simulink model "bu_abslut125_romvect_float"  (R2021b)
(part 3 of 8)

  AddSub121/1 -> Mux119/3
  Delay489/1 -> Relational184/1, Delay492/1
  AddSub163/1 -> Mux170/3
  Mux144/1 -> AddSub148/1, Delay376/1
  Delay586/1 -> Mux114/2
  Delay397/1 -> Mux160/1
  Delay542/1 -> Mux124/2
  Mux126/1 -> AddSub183/1, Delay245/1
  Delay529/1 -> Mux181/2
  Delay525/1 -> Mux169/2
  Delay550/1 -> Mux127/2
  Delay354/1 -> Mux152/2
  Delay248/1 -> Mux141/2
  Relational154/1 -> Delay350/1
  Relational199/1 -> Delay442/1
  AddSub181/1 -> Mux178/3
  Delay458/1 -> Mux102/1
  Mux95/1 -> AddSub99/1, Delay209/1
  Delay377/1 -> Delay378/1, Relational148/1
  Delay388/1 -> Relational160/1, Delay344/1
  AddSub124/1 -> Mux122/3
  Relational189/1 -> Delay504/1
  logi_b69/1 -> Relational145/2, Relational151/2
  Delay362/1 -> Mux154/2
  Delay378/1 -> Delay381/1, Relational149/1
  Delay473/1 -> Mux183/1
  AddSub188/1 -> Mux187/3
  Delay423/1 -> Mux163/2
  AddSub98/1 -> Mux95/3
  Mux162/1 -> AddSub165/1, Delay491/1
  Mux173/1 -> AddSub176/1, Delay469/1
  logi_b75/1 -> Relational153/2, Relational159/2
  Delay428/1 -> Relational101/1, Delay432/1
  Relational150/1 -> Delay386/1
  Delay480/1 -> Mux177/2
  Delay585/1 -> Mux114/1
  logi_b78/1 -> Relational177/2, Relational192/2
  Delay570/1 -> Delay573/1, Relational136/1
  Mux182/1 -> AddSub192/1, Delay411/1
  AddSub195/1 -> Mux163/3
  Relational115/1 -> Delay590/1
  Relational137/1 -> Delay578/1
  Relational185/1 -> Delay446/1
  Delay517/1 -> Mux120/2
  logi_b71/1 -> Relational147/2, Relational155/2
  Delay590/1 -> Mux115/1
  Delay210/1 -> Mux130/1
  Mux153/1 -> AddSub156/1, Delay362/1
  Delay415/1 -> Delay436/1, Relational197/1
  Delay511/1 -> Relational167/1, Delay514/1
  Delay484/1 -> Mux183/2
  Delay492/1 -> Relational186/1, Delay496/1
  Relational171/1 -> Delay527/1
  Delay557/1 -> Mux95/1
  AddSub106/1 -> Mux102/3
  Delay358/1 -> Mux153/2
  Delay589/1 -> Delay592/1, Relational116/1
  Relational174/1 -> Delay429/1
  Delay350/1 -> Mux151/1
  AddSub200/1 -> Mux197/3
  Delay420/1 -> Delay424/1, Relational200/1
  logi_b76/1 -> Relational160/2, Relational161/2
  Relational151/1 -> Delay340/1
  logi_b70/1 -> Relational146/2, Relational154/2
  AddSub107/1 -> Mux103/3
  logi_b67/1 -> Relational140/2, Relational142/2
  Delay367/1 -> Mux156/1
  Mux168/1 -> AddSub171/1, Delay525/1
  AddSub154/1 -> Mux149/3
  Relational146/1 -> Delay372/1
  Delay442/1 -> Mux197/1
  Mux133/1 -> AddSub135/1, Delay572/1
  Delay414/1 -> Mux193/2
  Mux170/1 -> AddSub173/1, Delay419/1
  Relational147/1 -> Delay375/1
  Mux104/1 -> AddSub101/1, Delay558/1
  AddSub180/1 -> Mux190/3
  Mux192/1 -> Delay418/1, AddSub104/1
  Mux113/1 -> AddSub117/1, Delay586/1
  AddSub134/1 -> Mux133/3
  Delay583/1 -> Mux113/2
  Delay569/1 -> Mux133/2
  AddSub118/1 -> Mux115/3
  Relational176/1 -> Delay487/1
  Delay559/1 -> Relational132/1, Delay562/1
  Mux131/1 -> AddSub132/1, Delay564/1
  Delay457/1 -> Relational175/1, Delay460/1
  Relational112/1 -> Delay224/1
  Delay436/1 -> Relational198/1, Delay441/1
  Delay394/1 -> Mux164/2
  Relational133/1 -> Delay563/1
  Delay591/1 -> Mux115/2
  Delay500/1 -> Delay503/1, Relational189/1
  Delay496/1 -> Delay497/1, Relational187/1
  Delay587/1 -> Delay589/1, Relational115/1
  AddSub136/1 -> Mux135/3
  logi_b92/1 -> Relational173/2, Relational190/2
  Delay515/1 -> Mux167/1
  Delay459/1 -> Mux102/2
  Relational162/1 -> Delay402/1
  Relational144/1 -> Delay332/1
  Mux187/1 -> AddSub189/1, Delay505/1
  Delay488/1 -> Mux162/2
  Delay223/1 -> Delay581/1, Relational112/1
  Relational113/1 -> Delay582/1
  AddSub123/1 -> Mux121/3
  Delay467/1 -> Relational178/1, Delay470/1
  Mux156/1 -> AddSub160/1, Delay343/1
  Delay222/1 -> Delay547/1, Relational37/1
  Delay553/1 -> Mux119/1
  Delay594/1 -> Mux116/2
  Delay439/1 -> Relational196/1, Delay462/1
  Relational193/1 -> Delay406/1
  AddSub116/1 -> Mux113/3
  Delay592/1 -> Delay595/1, Relational117/1
  Relational121/1 -> Delay553/1
  Relational130/1 -> Delay588/1
  Relational136/1 -> Delay574/1
  Delay462/1 -> Relational122/1, Delay495/1
  Mux197/1 -> AddSub138/1, Delay234/1
  Mux184/1 -> AddSub185/1, Delay494/1
  Mux130/1 -> AddSub141/1, Delay253/1
  Mux146/1 -> AddSub151/1, Delay384/1
  Mux191/1 -> Delay414/1, AddSub197/1
  Delay573/1 -> Relational137/1, Delay576/1
  Delay519/1 -> Mux170/1
  Delay334/1 -> Delay370/1, Relational145/1
  Relational145/1 -> Delay335/1
  AddSub133/1 -> Mux130/3
  Delay544/1 -> Mux125/1
  AddSub127/1 -> Mux125/3
  logi_b80/1 -> Relational179/2, Relational102/2
  Delay478/1 -> Relational183/1, Delay481/1
  logi_b51/1 -> Relational130/2, Relational124/2
  Delay497/1 -> Delay500/1, Relational188/1
  AddSub139/1 -> Mux150/3
  Relational129/1 -> Delay544/1
  AddSub140/1 -> Mux138/3
  Mux132/1 -> AddSub134/1, Delay569/1
  Mux135/1 -> AddSub137/1, Delay579/1
  AddSub165/1 -> Mux184/3
  Mux112/1 -> AddSub116/1, Delay583/1
  Mux127/1 -> Delay226/1, AddSub194/1
  logi_b86/1 -> Relational166/2, Relational172/2
  Delay402/1 -> Mux103/1
  Relational172/1 -> Delay400/1
  Delay386/1 -> Mux148/1
  Relational106/1 -> Delay458/1
  Delay363/1 -> Relational159/1, Delay366/1
  Mux151/1 -> AddSub153/1, Delay354/1
  AddSub147/1 -> Mux144/3
  Delay477/1 -> Mux176/2
  AddSub144/1 -> Mux151/3
  Relational138/1 -> Delay231/1
  AddSub172/1 -> Mux183/3
  Delay430/1 -> Mux200/1
  Delay422/1 -> Delay439/1, Relational185/1
  AddSub149/1 -> Mux146/3
  Constant2/1 -> AddSub31/2, AddSub9/2, AddSub11/2, AddSub33/2, AddSub35/2, AddSub36/2, AddSub37/2, AddSub60/2, AddSub44/2, AddSub52/2, AddSub54/2, AddSub55/2, AddSub56/2, AddSub59/2, AddSub79/2, AddSub112/2, AddSub63/2, AddSub81/2, AddSub83/2, AddSub84/2, AddSub85/2, AddSub109/2, AddSub130/2, AddSub194/2, AddSub105/2, AddSub132/2, AddSub134/2, AddSub135/2, AddSub136/2, AddSub162/2, AddSub144/2, AddSub153/2, AddSub155/2, AddSub156/2, AddSub157/2, AddSub160/2, AddSub182/2, AddSub113/2, AddSub165/2, AddSub185/2, AddSub187/2, AddSub188/2, AddSub189/2, AddSub104/2, AddSub196/2, AddSub238/2, AddSub205/2, AddSub294/2, AddSub293/2, AddSub207/2, AddSub291/2, AddSub288/2, AddSub287/2, AddSub286/2, AddSub285/2, AddSub283/2, AddSub263/2, AddSub262/2, AddSub211/2, AddSub280/2, AddSub209/2, AddSub206/2, AddSub299/2, AddSub289/2, AddSub278/2, AddSub271/2, AddSub261/2, AddSub258/2, AddSub256/2, AddSub255/2, AddSub254/2, AddSub140/2, AddSub102/2, AddSub195/2, AddSub193/2, AddSub190/2, AddSub164/2, AddSub106/2, AddSub103/2, AddSub201/2, AddSub191/2, AddSub180/2, AddSub173/2, AddSub163/2, AddSub158/2, AddSub143/2, AddSub142/2, AddSub137/2, AddSub101/2, AddSub172/2, AddSub161/2, AddSub150/2, AddSub139/2, AddSub128/2, AddSub120/2, AddSub99/2, AddSub98/2, AddSub40/2, AddSub100/2, AddSub91/2, AddSub90/2, AddSub89/2, AddSub86/2, AddSub62/2, AddSub110/2, AddSub108/2, AddSub97/2, AddSub87/2, AddSub77/2, AddSub70/2, AddSub61/2, AddSub57/2, AddSub43/2, AddSub42/2, AddSub38/2, AddSub10/2, AddSub7/2, AddSub6/2, AddSub5/2, AddSub4/2, AddSub3/2, AddSub2/2, AddSub1/2, AddSub/2, Mux/3
  Delay522/1 -> Mux168/2
  Delay441/1 -> Relational199/1, Delay444/1
  Delay333/1 -> Mux142/2
  Delay244/1 -> Relational38/1, Delay552/1
  AddSub299/1 -> Mux204/3
  logi_b110/1 -> Relational262/2, Relational275/2
  logi_b109/1 -> Relational283/2, Relational210/2
  Delay726/1 -> Relational238/1
  Relational259/1 -> Delay661/1
  Delay747/1 -> Mux204/2
  Relational264/1 -> Delay691/1
  AddSub291/1 -> Mux292/3
  Delay734/1 -> Mux296/2
  Delay760/1 -> Mux273/2
  AddSub205/1 -> Mux300/3
  Delay624/1 -> Mux249/1
  Delay758/1 -> Relational277/1, Delay761/1
  AddSub250/1 -> Mux248/3
  Relational206/1 -> Delay742/1
  Delay613/1 -> Mux237/1
  Delay718/1 -> Relational302/1, Delay722/1
  Mux281/1 -> AddSub284/1, Delay685/1
  AddSub288/1 -> Mux289/3
  Relational283/1 -> Delay776/1
  logi_b120/1 -> Relational295/2, Relational294/2
  logi_b121/1 -> Relational297/2, Relational300/2
  Delay662/1 -> Mux256/2
  Relational292/1 -> Delay703/1
  Delay763/1 -> Mux274/2
  AddSub267/1 -> Mux267/3
  Delay658/1 -> Mux255/1
  Delay432/1 -> Relational138/1, Delay610/1
  Delay715/1 -> Mux263/1
  Delay705/1 -> Mux291/2
  Relational290/1 -> Delay802/1
  Delay785/1 -> Mux284/2
  logi_b115/1 -> Relational269/2, Relational287/2
  Mux286/1 -> AddSub286/1, Delay796/1
  Delay787/1 -> Mux285/1
  Delay814/1 -> Delay817/1, Relational270/1
  AddSub249/1 -> Mux247/3
  Delay737/1 -> Mux297/2
  AddSub282/1 -> Mux281/3
  Delay721/1 -> Mux299/2
  Delay625/1 -> Mux249/2
  logi_b105/1 -> Relational278/2, Relational301/2
  Delay788/1 -> Mux285/2
  AddSub262/1 -> Mux262/3
  AddSub269/1 -> Mux269/3
  AddSub264/1 -> Mux264/3
  Mux263/1 -> AddSub294/1, Delay721/1
  Relational203/1 -> Delay655/1
  Delay700/1 -> Mux292/1
  Mux258/1 -> Delay683/1, AddSub261/1
  Delay704/1 -> Mux291/1
  Mux204/1 -> AddSub206/1, Delay750/1
  Delay765/1 -> Delay769/1, Relational280/1
  Relational287/1 -> Delay792/1
  Delay701/1 -> Mux292/2
  Mux271/1 -> AddSub273/1, Delay760/1
  Mux277/1 -> AddSub279/1, Delay777/1
  Relational301/1 -> Delay727/1
  logi_b111/1 -> Relational265/2, Relational264/2
  Delay697/1 -> Mux207/2
  Delay711/1 -> Mux259/1
  Relational288/1 -> Delay795/1
  Delay817/1 -> Delay820/1, Relational271/1
  Delay659/1 -> Mux255/2
  Delay739/1 -> Delay741/1, Relational206/1
  Delay803/1 -> Mux289/2
  Relational295/1 -> Delay706/1
  Delay712/1 -> Mux259/2
  AddSub297/1 -> Mux296/3
  Mux254/1 -> AddSub255/1, Delay659/1
  Delay614/1 -> Mux237/2
  Relational253/1 -> Delay624/1
  AddSub256/1 -> Mux256/3
  Delay764/1 -> Delay765/1, Relational279/1
  Delay713/1 -> Mux280/2
  Delay780/1 -> Relational265/1, Delay689/1
  Delay660/1 -> Relational261/1, Delay635/1
  Mux260/1 -> AddSub262/1, Delay782/1
  Mux290/1 -> AddSub289/1, Delay743/1
  Relational286/1 -> Delay787/1
  AddSub283/1 -> Mux285/3
  Mux300/1 -> AddSub238/1, Delay612/1
  Delay679/1 -> Relational253/1, Delay682/1
  AddSub285/1 -> Mux286/3
  Delay807/1 -> Mux266/2
  Delay798/1 -> Mux288/1
  Delay684/1 -> Mux282/1
  Relational302/1 -> Delay720/1
  Delay762/1 -> Mux274/1
  Relational268/1 -> Delay809/1
  Delay703/1 -> Mux280/1
  AddSub272/1 -> Mux271/3
  Delay812/1 -> Delay814/1, Relational269/1
  Mux205/1 -> AddSub209/1, Delay753/1
  Delay821/1 -> Mux281/1
  AddSub254/1 -> Mux254/3
  Mux206/1 -> AddSub280/1, Delay779/1
  Relational277/1 -> Delay759/1
  Relational284/1 -> Delay784/1
  AddSub277/1 -> Mux277/3
  Delay775/1 -> Relational262/1, Delay780/1
  Delay444/1 -> Relational139/1, Delay617/1
  AddSub289/1 -> Mux298/3
  Mux259/1 -> AddSub293/1, Delay717/1
  Mux249/1 -> AddSub257/1, Delay640/1
  Delay799/1 -> Mux288/2
  logi_b119/1 -> Relational291/2, Relational293/2
  Relational278/1 -> Delay762/1
  Delay742/1 -> Mux298/1
  AddSub294/1 -> Mux299/3
  Relational208/1 -> Delay749/1
  Relational291/1 -> Delay704/1
  Delay640/1 -> Mux257/2
  Relational275/1 -> Delay755/1
  Delay719/1 -> Relational301/1, Delay739/1
  Mux257/1 -> Delay757/1, AddSub272/1
  Delay749/1 -> Mux205/1
  AddSub273/1 -> Mux273/3
  Delay741/1 -> Delay744/1, Relational207/1
  Delay796/1 -> Mux287/2
  logi_b103/1 -> Relational276/2, Relational282/2
  AddSub211/1 -> Mux260/3
  logi_b113/1 -> Relational267/2, Relational284/2
  Delay804/1 -> Mux265/2
  AddSub284/1 -> Mux282/3
  Delay776/1 -> Mux278/1
  Delay797/1 -> Relational290/1, Delay801/1
  Relational204/1 -> Delay677/1
  Delay681/1 -> Mux248/2
  AddSub274/1 -> Mux274/3
  AddSub268/1 -> Mux268/3
  Delay766/1 -> Mux275/1
  Relational260/1 -> Delay639/1
  AddSub257/1 -> Mux257/3
  AddSub275/1 -> Mux275/3
  Relational298/1 -> Delay732/1
  Delay781/1 -> Mux271/1
  Delay770/1 -> Mux276/1
  Delay746/1 -> Mux204/1
  Delay738/1 -> Relational239/1
  Relational300/1 -> Delay715/1
  Delay743/1 -> Mux298/2
  Relational266/1 -> Delay690/1
  Delay748/1 -> Relational210/1, Delay751/1
  Delay677/1 -> Mux247/1
  Mux276/1 -> AddSub277/1, Delay774/1
  Mux269/1 -> AddSub282/1, Delay823/1
  Delay801/1 -> Relational293/1, Delay699/1
  Relational297/1 -> Delay710/1
  Mux248/1 -> AddSub252/1, Delay625/1
  Delay754/1 -> Relational264/1, Delay693/1
  Relational265/1 -> Delay686/1
  Delay769/1 -> Delay772/1, Relational281/1
  Delay777/1 -> Mux278/2
  Delay612/1 -> Mux238/2
  Mux207/1 -> Delay688/1, AddSub264/1
  Mux289/1 -> AddSub291/1, Delay701/1
  Delay824/1 -> Relational291/1, Delay702/1
  logi_b117/1 -> Relational271/2, Relational289/2
  Mux293/1 -> AddSub296/1, Delay729/1
  logi_b108/1 -> Relational281/2, Relational208/2
  Mux280/1 -> AddSub278/1, Delay731/1
  Mux285/1 -> AddSub285/1, Delay793/1
  Delay639/1 -> Mux257/1
  AddSub265/1 -> Mux265/3
  logi_b116/1 -> Relational270/2, Relational288/2
  Mux288/1 -> AddSub288/1, Delay803/1
  AddSub276/1 -> Mux276/3
  Delay802/1 -> Mux289/1
  Delay720/1 -> Mux299/1
  Delay706/1 -> Mux293/1
  Relational207/1 -> Delay746/1
  Delay725/1 -> Mux300/2
  Delay686/1 -> Mux264/1
  Mux295/1 -> AddSub297/1, Delay734/1
  Delay699/1 -> Relational294/1, Delay714/1
  Delay727/1 -> Mux290/1
  Delay795/1 -> Mux287/1
  Relational239/1 -> Delay613/1
  Mux267/1 -> AddSub268/1, Delay816/1
  Delay759/1 -> Mux273/1
  Delay611/1 -> Mux238/1
  Delay773/1 -> Mux277/1
  AddSub236/1 -> Mux237/3
  AddSub255/1 -> Mux255/3
  Delay744/1 -> Delay748/1, Relational208/1
  Delay779/1 -> Mux279/2
  Mux298/1 -> AddSub299/1, Delay747/1
  logi_b124/1 -> Relational239/2, Relational238/2
  Relational280/1 -> Delay770/1
  Delay638/1 -> Delay758/1, Relational276/1
  Delay694/1 -> Mux262/1
  Delay689/1 -> Delay805/1, Relational266/1
  Delay808/1 -> Relational268/1, Delay812/1
  Mux296/1 -> AddSub298/1, Delay737/1
  Mux255/1 -> AddSub256/1, Delay662/1
  AddSub206/1 -> Mux205/3
  Delay693/1 -> Delay783/1, Relational272/1
  Delay695/1 -> Relational292/1, Delay719/1
  Delay793/1 -> Mux286/2
  Delay768/1 -> Mux275/2
  Relational282/1 -> Delay813/1
  Delay755/1 -> Mux279/1
  Delay792/1 -> Mux286/1
  Delay683/1 -> Mux270/2
  Delay655/1 -> Mux254/1
  Mux279/1 -> Delay692/1, AddSub211/1
  Delay710/1 -> Mux295/1
  Delay757/1 -> Mux271/2
  Delay637/1 -> Mux258/2
  Mux247/1 -> AddSub250/1, Delay681/1
  Delay784/1 -> Mux284/1
  Delay690/1 -> Mux265/1
  Mux265/1 -> AddSub266/1, Delay807/1
  AddSub266/1 -> Mux266/3
  Mux299/1 -> AddSub205/1, Delay725/1
  AddSub296/1 -> Mux295/3
  Delay815/1 -> Mux268/1
  logi_b123/1 -> Relational299/2, Relational205/2
  Relational258/1 -> Delay658/1
  Relational267/1 -> Delay806/1
  Relational279/1 -> Delay766/1
  AddSub290/1 -> Mux291/3
  Delay729/1 -> Mux295/2
  Delay731/1 -> Mux290/2
  Delay806/1 -> Mux266/1
  Delay692/1 -> Mux260/2
  logi_b122/1 -> Relational298/2, Relational302/2
  Mux278/1 -> AddSub210/1, Delay697/1
  AddSub280/1 -> Mux279/3
  Delay636/1 -> Mux258/1
  Relational270/1 -> Delay818/1
  Relational281/1 -> Delay773/1
  Relational269/1 -> Delay815/1
  AddSub271/1 -> Mux280/3
  AddSub258/1 -> Mux258/3
  Mux264/1 -> AddSub265/1, Delay804/1
  AddSub295/1 -> Mux293/3
  Relational294/1 -> Delay711/1
  Delay818/1 -> Mux269/1
  Delay702/1 -> Relational295/1, Delay709/1
  Delay810/1 -> Mux267/2
  logi_b107/1 -> Relational280/2, Relational207/2
  AddSub207/1 -> Mux259/3
  Delay685/1 -> Mux282/2
  Relational205/1 -> Delay724/1
  Delay750/1 -> Mux205/2
  logi_b114/1 -> Relational268/2, Relational286/2
  Delay732/1 -> Mux296/1
  Delay678/1 -> Mux247/2
  Relational261/1 -> Delay636/1
  Mux275/1 -> AddSub276/1, Delay771/1
  Relational273/1 -> Delay684/1
  Delay820/1 -> Relational273/1, Delay824/1
  Delay635/1 -> Delay695/1, Relational282/1
  Mux266/1 -> AddSub267/1, Delay810/1
  logi_b100/1 -> Relational250/2, Relational258/2
  AddSub287/1 -> Mux288/3
  Mux274/1 -> AddSub275/1, Delay768/1
  Delay783/1 -> Relational284/1, Delay786/1
  AddSub261/1 -> Mux270/3
  Delay691/1 -> Mux260/1
  Delay823/1 -> Mux281/2
  Delay819/1 -> Mux269/2
  Relational299/1 -> Delay736/1
  AddSub279/1 -> Mux278/3
  Delay752/1 -> Mux206/1
  Delay682/1 -> Relational260/1, Delay638/1
  Relational289/1 -> Delay798/1
  Delay656/1 -> Mux254/2
  AddSub286/1 -> Mux287/3
  Delay717/1 -> Mux263/2
  Mux262/1 -> AddSub263/1, Delay785/1
  Mux273/1 -> AddSub274/1, Delay763/1
  logi_b101/1 -> Relational253/2, Relational259/2
  Delay722/1 -> Relational205/1, Delay726/1
  Relational250/1 -> Delay680/1
  Delay774/1 -> Mux277/2
  logi_b104/1 -> Relational277/2, Relational292/2
  Mux282/1 -> AddSub290/1, Delay705/1
  AddSub293/1 -> Mux263/3
  Delay709/1 -> Delay730/1, Relational297/1
  Delay805/1 -> Relational267/1, Delay808/1
  Delay786/1 -> Relational286/1, Delay790/1
  Relational271/1 -> Delay821/1
  AddSub209/1 -> Mux206/3
  AddSub298/1 -> Mux297/3
  Delay714/1 -> Delay718/1, Relational300/1
  logi_b102/1 -> Relational260/2, Relational261/2
  AddSub210/1 -> Mux207/3
  Delay661/1 -> Mux256/1
  Mux268/1 -> AddSub269/1, Delay819/1
  AddSub252/1 -> Mux249/3
  Delay736/1 -> Mux297/1
  Delay708/1 -> Mux293/2
  Mux270/1 -> AddSub271/1, Delay713/1
  AddSub278/1 -> Mux290/3
  Mux292/1 -> Delay712/1, AddSub207/1
  Relational276/1 -> Delay781/1
  Delay751/1 -> Relational275/1, Delay754/1
  Delay730/1 -> Relational298/1, Delay735/1
  Delay688/1 -> Mux264/2
  Delay794/1 -> Delay797/1, Relational289/1
  Delay790/1 -> Delay791/1, Relational287/1
  logi_b118/1 -> Relational273/2, Relational290/2
  Delay809/1 -> Mux267/1
  Delay753/1 -> Mux206/2
  Relational262/1 -> Delay696/1
  Mux287/1 -> AddSub287/1, Delay799/1
  Delay782/1 -> Mux262/2
  Delay761/1 -> Relational278/1, Delay764/1
  Mux256/1 -> AddSub258/1, Delay637/1
  Relational293/1 -> Delay700/1
  Mux297/1 -> AddSub236/1, Delay614/1
  Mux284/1 -> AddSub283/1, Delay788/1
  Mux291/1 -> Delay708/1, AddSub295/1
  Delay813/1 -> Mux270/1
  logi_b106/1 -> Relational279/2, Relational206/2
  Delay772/1 -> Relational283/1, Delay775/1
  Delay791/1 -> Delay794/1, Relational288/1
  AddSub238/1 -> Mux238/3
  AddSub263/1 -> Mux284/3
  logi_b112/1 -> Relational266/2, Relational272/2
  Delay696/1 -> Mux207/1
  Relational272/1 -> Delay694/1
  Delay680/1 -> Mux248/1
  Relational210/1 -> Delay752/1
  Delay657/1 -> Relational259/1, Delay660/1
  Delay771/1 -> Mux276/2
  Relational238/1 -> Delay611/1
  Delay724/1 -> Mux300/1
  Delay816/1 -> Mux268/2
  Delay735/1 -> Relational299/1, Delay738/1
  Mux237/1 -> Slice1/1
  Mux138/1 -> AddSub254/1, Delay656/1
  logi_b99/1 -> Relational204/2, Relational203/2
  Mux137/1 -> AddSub249/1, Delay678/1
  Delay547/1 -> Relational95/1, Delay577/1
  Mux238/1 -> Slice/1
  ROM3/1 -> Mux93/5
  ROM4/1 -> Mux93/6
  ROM5/1 -> Mux93/7
  ROM6/1 -> Mux93/8
  ROM7/1 -> Mux93/9
  Delay599/1 -> ROM3/1
  Delay600/1 -> ROM4/1
  Delay601/1 -> ROM5/1
  Delay602/1 -> ROM6/1
  Delay603/1 -> ROM7/1
  Constant10/1 -> Relational119/2
  AddSub96/1 -> AddSub202/1
  Relational119/1 -> AddSub202/2
  Constant11/1 -> Relational123/2
  AddSub202/1 -> AddSub203/1
  Relational123/1 -> AddSub203/2
  Constant12/1 -> Relational209/2
  AddSub203/1 -> AddSub204/1
  Relational209/1 -> AddSub204/2
  Constant13/1 -> Relational211/2
  AddSub204/1 -> AddSub208/1
  Relational211/1 -> AddSub208/2
  Constant14/1 -> Relational212/2
  AddSub208/1 -> AddSub212/1
  Relational212/1 -> AddSub212/2
  Slice3/1 -> Delay198/1, Delay603/1, Delay602/1, Delay601/1, Delay600/1, Delay599/1, Delay208/1, Delay197/1, Delay609/1, Delay605/1, Relational94/1, Relational93/1, Delay606/1, Delay607/1, Delay608/1
  AddSub212/1 -> Mux93/1
  Gateway Out/1 -> Output/1
  Constant5/1 -> Delay604/1
  Delay605/1 -> Relational119/1
  Delay606/1 -> Relational123/1
  Delay607/1 -> Relational209/1
  Delay608/1 -> Relational211/1
  Delay609/1 -> Relational212/1
  Delay604/1 -> AddSub22/2
  Slice/1 -> Gateway Out1/1, Delay60/1, AddSub18/1, Delay59/1
  Slice1/1 -> Delay61/1, Gateway Out2/1
  Gateway Out1/1 -> To Workspace3/1
  Gateway Out2/1 -> To Workspace1/1
  Delay610/1 -> Relational203/1, Delay615/1
  Delay615/1 -> Relational258/1, Delay657/1
  Delay616/1 -> Relational250/1, Delay679/1
  Delay617/1 -> Relational204/1, Delay616/1
